simulink model "lorenz_sim"  (R2024a)
settings: Solver=ode4  StartTime=0.0  StopTime=100  FixedStep=0.001  RelTol=1e-3
PreLoadFcn:
  | sigma = 10; rho = 28; beta = 8/3;
  | x0 = 1; y0 = 1; z0 = 1;
  | assignin('base', 'sigma', sigma);
  | assignin('base', 'rho',   rho);
  | assignin('base', 'beta',  beta);
  | assignin('base', 'x0',    x0);
  | assignin('base', 'y0',    y0);
  | assignin('base', 'z0',    z0);
StopFcn:
  | plot_lorenz_attractor
settings Model: Creator=javie  LastModifiedBy=javie
settings DataIOCC: ReturnWorkspaceOutputs=off

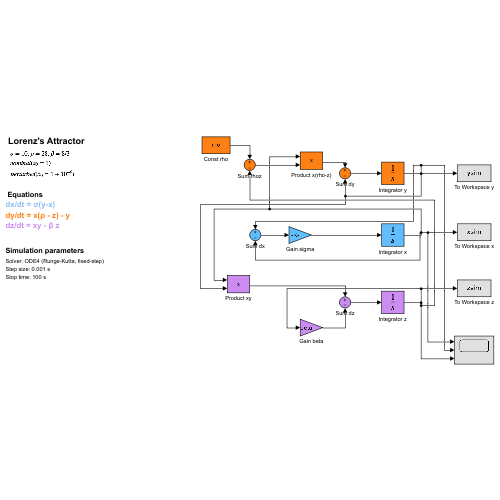
[thumbnail: Simulink's stored preview of the top-level diagram]
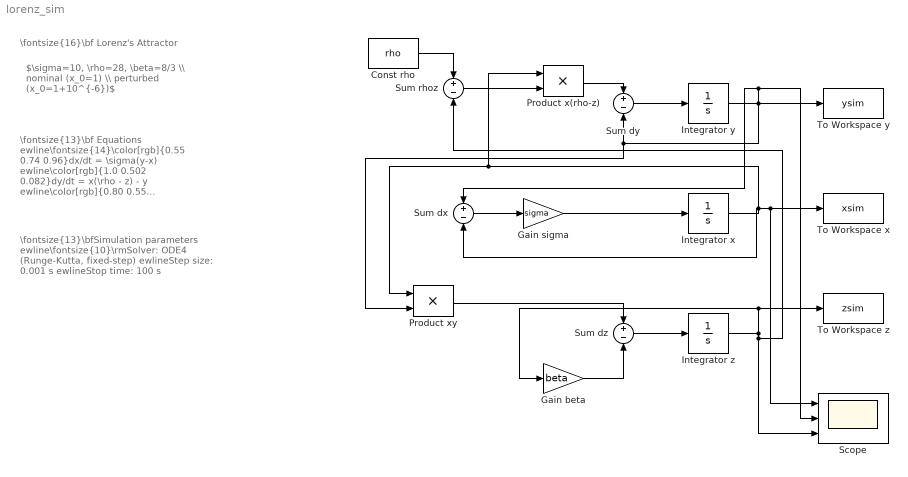
== system lorenz_sim ==
  note: $\sigma=10, \rho=28, \beta=8/3 \\ nominal (x_0=1) \\ perturbed (x_0=1+10^{-6})$
  note: \fontsize{16}\bf Lorenz's Attractor
  note: \fontsize{13}\bf Equations\newline\fontsize{14}\color[rgb]{0.55 0.74 0.96}dx/dt = \sigma(y-x)\newline\color[rgb]{1.0 0.502 0.082}dy/dt = x(\rho - z) - y\newline\color[rgb]{0.80 0.55 0.95}dz/dt = xy - \beta z
  note: \fontsize{13}\bfSimulation parameters\newline\fontsize{10}\rmSolver: ODE4 (Runge-Kutta, fixed-step)\newlineStep size: 0.001 s\newlineStop time: 100 s
  Const rho : Constant  Value=rho
  Gain beta : Gain  Gain=beta
  Gain sigma : Gain  Gain=sigma
  Integrator x : Integrator  InitialCondition=x0
  Integrator y : Integrator  InitialCondition=y0
  Integrator z : Integrator  InitialCondition=z0
  Product x(rho-z) : Product  Inputs=**
  Product xy : Product  Inputs=**
  Scope : Scope  NumInputPorts=3
  Sum dx : Sum  Inputs=+-
  Sum dy : Sum  Inputs=+-
  Sum dz : Sum  Inputs=+-
  Sum rhoz : Sum  Inputs=+-
  To Workspace x : ToWorkspace  VariableName=xsim  SaveFormat=Timeseries  SampleTime=-1
  To Workspace y : ToWorkspace  VariableName=ysim  SaveFormat=Timeseries  SampleTime=-1
  To Workspace z : ToWorkspace  VariableName=zsim  SaveFormat=Timeseries  SampleTime=-1
  wires:
  Sum dz/1 -> Integrator z/1
  Gain beta/1 -> Sum dz/2
  Product xy/1 -> Sum dz/1
  Sum dy/1 -> Integrator y/1
  Product x(rho-z)/1 -> Sum dy/1
  Sum rhoz/1 -> Product x(rho-z)/2
  Integrator z/1 -> To Workspace z/1, Gain beta/1, Scope/3, Sum rhoz/2
  Const rho/1 -> Sum rhoz/1
  Gain sigma/1 -> Integrator x/1
  Sum dx/1 -> Gain sigma/1
  Integrator x/1 -> Scope/1, To Workspace x/1, Product xy/1, Product x(rho-z)/1, Sum dx/2
  Integrator y/1 -> Product xy/2, Sum dy/2, To Workspace y/1, Scope/2, Sum dx/1
